simulink model "IS_Simulator"  (R2017a)
settings: Solver=VariableStepAuto  StartTime=0.0  StopTime=0.5  RelTol=1e-3
values from neighbouring files (symbols this model uses):
  A0 = 1/(1+2*K+K^2)    [InputShaper.m]
  A1 = 2*K/(1+2*K+K^2)    [InputShaper.m]
  A2 = K^2/(1+2*K+K^2)    [InputShaper.m]
  t1 = Td/2    (= 0.23)    [InputShaper.m]
  t2 = Td    (= 0.46)    [InputShaper.m]
libraries: cstblocks x2
settings Model: Creator=capn  LastModifiedBy=capn

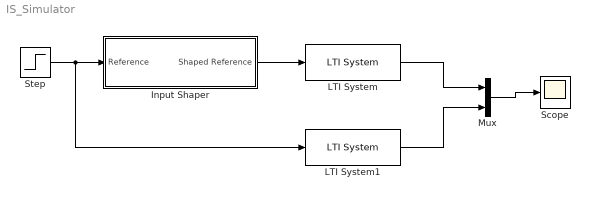
== system IS_Simulator ==
  Input Shaper : Subsystem
  LTI System : cstblocks/LTI System  sys=G  IC=[]
  LTI System1 : cstblocks/LTI System  sys=G  IC=[]
  Mux : Mux  Inputs=2
  Scope : Scope
  Step : Step  Time=0  SampleTime=0
  wires:
  Step/1 -> LTI System1/1, Input Shaper/1(Reference)
  Input Shaper/1(Shaped Reference) -> LTI System/1
  LTI System/1 -> Mux/1
  LTI System1/1 -> Mux/2
  Mux/1 -> Scope/1

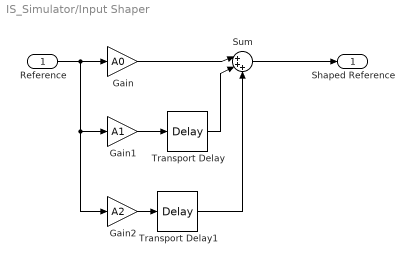
== system IS_Simulator/Input Shaper ==
  Reference : Inport
  Gain : Gain  Gain=A0
  Gain1 : Gain  Gain=A1
  Gain2 : Gain  Gain=A2
  Sum : Sum  Inputs=|+++
  Transport Delay : TransportDelay  DelayTime=t1
  Transport Delay1 : TransportDelay  DelayTime=t2
  Shaped Reference : Outport
  wires:
  Reference/1 -> Gain1/1, Gain2/1, Gain/1
  Gain/1 -> Sum/1
  Sum/1 -> Shaped Reference/1
  Gain1/1 -> Transport Delay/1
  Transport Delay/1 -> Sum/2
  Gain2/1 -> Transport Delay1/1
  Transport Delay1/1 -> Sum/3
